simulink model "simulink_disturbio"  (R2021a)
settings: Solver=VariableStepAuto  StartTime=0.0  StopTime=130  RelTol=1e-3
values from neighbouring files (symbols this model uses):
  F_C2 = (1 - pos_pf2) / (z - pos_pf2)    [Q1_C.m]
  Ts = tsd/25    [Q1_A.m]    (also in Q1_B.m; Q1_C.m; Q2_AB.m = 0.76; Q2_C.m = 0.76)
settings Model: Creator=ribei  LastModifiedBy=check
settings SolverCC: AlgebraicLoopSolver=TrustRegion
settings DebuggingCC: UnconnectedInputMsg=none  UnconnectedOutputMsg=none  UnconnectedLineMsg=none  SFMachineParentedDataDiag=warning  ArithmeticOperatorsInVariantConditions=warning
settings ModelReferenceCC: EnableRefExpFcnMdlSchedulingChecks=off
settings SFSimCC: CustomCodeUndefinedFunction=UseInterfaceOnly
settings RTWCC: Description=Generic Real-Time Target
settings CodeAppCC: StateflowObjectComments=on

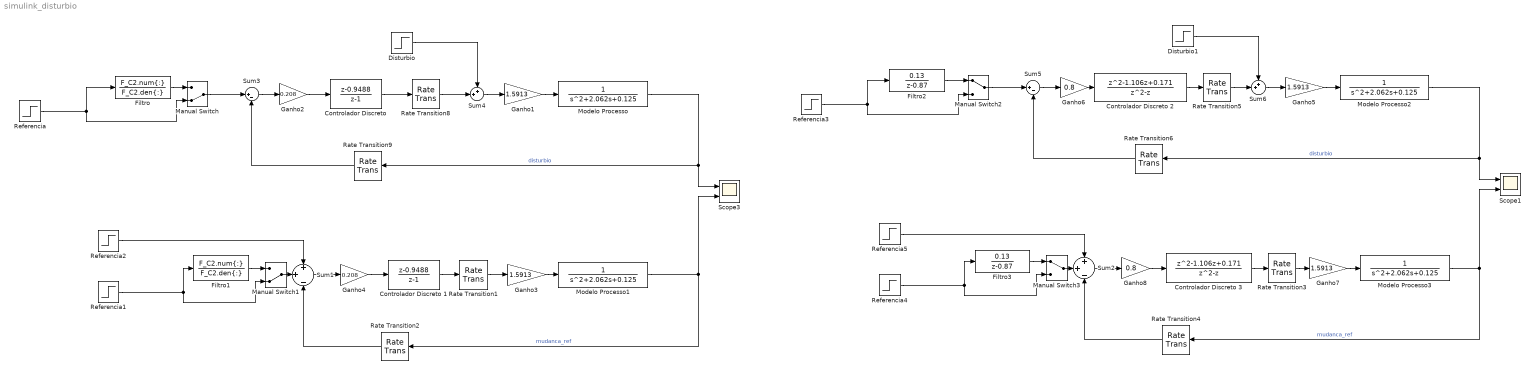
== system simulink_disturbio ==
  "Controlador Discreto " : DiscreteTransferFcn  Numerator=[1 -0.9488]  Denominator=[1 -1]
  Controlador Discreto 1 : DiscreteTransferFcn  Numerator=[1 -0.9488]  Denominator=[1 -1]
  Controlador Discreto 2 : DiscreteTransferFcn  Numerator=[1 -1.106 0.171]  Denominator=[1 -1 0]
  Controlador Discreto 3 : DiscreteTransferFcn  Numerator=[1 -1.106 0.171]  Denominator=[1 -1 0]
  Disturbio : Step  Time=35  SampleTime=Ts  VectorParams1D=off
  Disturbio1 : Step  Time=35  SampleTime=Ts  VectorParams1D=off
  Filtro : DiscreteTransferFcn  Numerator=F_C2.num{:}  Denominator=F_C2.den{:}
  Filtro1 : DiscreteTransferFcn  Numerator=F_C2.num{:}  Denominator=F_C2.den{:}
  Filtro2 : DiscreteTransferFcn  Numerator=[0.13]  Denominator=[1 -0.87]
  Filtro3 : DiscreteTransferFcn  Numerator=[0.13]  Denominator=[1 -0.87]
  Ganho{1,3,5,7} (4 alike) : Gain  Gain=1.5913
  Ganho2 : Gain  Gain=0.208
  Ganho4 : Gain  Gain=0.208
  Ganho6 : Gain  Gain=0.8
  Ganho8 : Gain  Gain=0.8
  Manual Switch : ManualSwitch  CurrentSetting=0
  Manual Switch1 : ManualSwitch  CurrentSetting=0
  Manual Switch2 : ManualSwitch
  Manual Switch3 : ManualSwitch
  Modelo Processo{,1..3} (4 alike) : TransferFcn  Denominator=[1 2.062 0.125]
  Rate Transition{1,3,5,8} (4 alike) : RateTransition  Integrity=off  OutPortSampleTimeOpt=Inherit
  Rate Transition{2,4,6,9} (4 alike) : RateTransition  OutPortSampleTime=Ts
  Referencia{,1,3..4} (4 alike) : Step  SampleTime=Ts
  Referencia2 : Step  Time=35  SampleTime=Ts
  Referencia5 : Step  Time=35  SampleTime=Ts
  Scope1 : Scope  NumInputPorts=2
  Scope3 : Scope  NumInputPorts=2
  Sum1 : Sum  Inputs=+|+|-
  Sum2 : Sum  Inputs=+|+|-
  Sum3 : Sum  Inputs=|+-
  Sum4 : Sum  Inputs=++|
  Sum5 : Sum  Inputs=|+-
  Sum6 : Sum  Inputs=++|
  wires:
  Disturbio/1 -> Sum4/1
  Referencia/1 -> Manual Switch/2, Filtro/1
  Sum3/1 -> Ganho2/1
  Modelo Processo/1 -> Rate Transition9/1, Scope3/1  "disturbio"
  Rate Transition9/1 -> Sum3/2
  "Controlador Discreto "/1 -> Rate Transition8/1
  Rate Transition8/1 -> Sum4/2
  Manual Switch/1 -> Sum3/1
  Filtro/1 -> Manual Switch/1
  Controlador Discreto 1/1 -> Rate Transition1/1
  Rate Transition2/1 -> Sum1/3
  Modelo Processo1/1 -> Scope3/2, Rate Transition2/1  "mudanca_ref"
  Referencia1/1 -> Manual Switch1/2, Filtro1/1
  Filtro1/1 -> Manual Switch1/1
  Manual Switch1/1 -> Sum1/2
  Referencia2/1 -> Sum1/1
  Ganho2/1 -> "Controlador Discreto "/1
  Ganho1/1 -> Modelo Processo/1
  Sum4/1 -> Ganho1/1
  Ganho3/1 -> Modelo Processo1/1
  Rate Transition1/1 -> Ganho3/1
  Ganho4/1 -> Controlador Discreto 1/1
  Sum1/1 -> Ganho4/1
  Sum2/1 -> Ganho8/1
  Ganho8/1 -> Controlador Discreto 3/1
  Rate Transition3/1 -> Ganho7/1
  Ganho7/1 -> Modelo Processo3/1
  Sum6/1 -> Ganho5/1
  Ganho5/1 -> Modelo Processo2/1
  Ganho6/1 -> Controlador Discreto 2/1
  Referencia5/1 -> Sum2/1
  Manual Switch3/1 -> Sum2/2
  Filtro3/1 -> Manual Switch3/1
  Referencia4/1 -> Filtro3/1, Manual Switch3/2
  Modelo Processo3/1 -> Rate Transition4/1, Scope1/2  "mudanca_ref"
  Rate Transition4/1 -> Sum2/3
  Controlador Discreto 3/1 -> Rate Transition3/1
  Filtro2/1 -> Manual Switch2/1
  Manual Switch2/1 -> Sum5/1
  Rate Transition5/1 -> Sum6/2
  Controlador Discreto 2/1 -> Rate Transition5/1
  Rate Transition6/1 -> Sum5/2
  Modelo Processo2/1 -> Scope1/1, Rate Transition6/1  "disturbio"
  Sum5/1 -> Ganho6/1
  Referencia3/1 -> Filtro2/1, Manual Switch2/2
  Disturbio1/1 -> Sum6/1
